simulink model "Power_Quality_Test2"  (R2015a)
settings: Solver=ode23t  StartTime=0.0  StopTime=0.5  RelTol=1e-5  AbsTol=1e-4
PreLoadFcn:
  | Ts=2e-6;
  | decimation = 1;
undefined symbols (not defined in the file or in its folder): HEV_Param
libraries: HEV_Electrical_Lib x5, fl_lib x2, simulink x1, HEV_Battery_Det_Lib x1, nesl_utility x1, powerlib x1
Description:
  | Copyright 2014 The MathWorks, Inc.
settings Model: CovSFcnEnable=off  Creator=smiller  LastModifiedBy=psanghvi
settings DataIOCC: SignalLoggingSaveFormat=ModelDataLogs
settings OptimizationCC: ExpressionDepthLimit=2147483647
settings DebuggingCC: UnderspecifiedInitializationDetection=Classic  MergeDetectMultiDrivingBlocksExec=none  SolverPrmCheckMsg=warning  FcnCallInpInsideContextMsg=UseLocalSettings  StateNameClashWarn=warning
settings SFSimCC: SimParseCustomCode=off
settings GRTTargetCC: CombineOutputUpdateFcns=off  GRTInterface=on

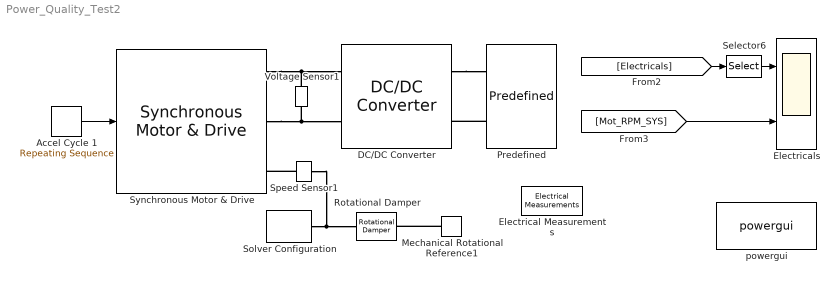
== system Power_Quality_Test2 ==
  Accel Cycle 1 : simulink/Sources/Repeating Sequence  rep_seq_t=[0 0.05 0.3 0.31 30]  rep_seq_y=[0 0.4 0.4 0.1 0.1]*100
  DC/DC Converter : HEV_Electrical_Lib/Detailed/DC//DC Converter  SystemSampleTime=-1
  Electrical Measurements : HEV_Electrical_Lib/Detailed/Electrical Measurements
  Electricals : Scope  NumInputPorts=2
      settings: YMin=499~200  YMax=501~500  SaveName=Electricals  Decimation=decimation
  Mechanical Rotational Reference1 : fl_lib/Mechanical/Rotational Elements/Mechanical Rotational Reference
  Predefined : HEV_Battery_Det_Lib/Predefined  SystemSampleTime=-1
  Rotational Damper : fl_lib/Mechanical/Rotational Elements/Rotational Damper  D=HEV_Param.ICE.Friction N*m/(rad/s)  w_specify=off  w_priority=High  w=0 rad/s  t_specify=off  t_priority=High  t=0 N*m
  Selector6 : Selector  InputPortWidth=8  Indices=[3 4]
  Solver Configuration : nesl_utility/Solver Configuration  PhysicalDomain=network_engine_domain  SubClassName=solver  LeftPortType=input  RightPortType=generic  Accelerate=off  Tones=[]  Harmonics=[]  SimulateNoise=off  Profile=off  UseLocalSampling=off  EnableSwitchedLinearOptims=on  FrequencyDomain=off  UseCCode=off  RelTol=0.001  AbsTol=1e-06  MinStep=1e-09  ToWorkspace=off  RevertToSquareIcSolve=off  NumHomotopyIterations=100  DoDC=off  ResidualTolerance=1e-9  UseLocalSolver=off  LocalSolverChoice=NE_BACKWARD_EULER_ADVANCER  LocalSolverSampleTime=.001  DoFixedCost=off  MaxNonlinIter=3  MaxModeIter=2  LinearAlgebra=Sparse  DelaysMemoryBudget=1024  AutomaticFiltering=on  FilteringTimeConstant=0.001
  Speed Sensor1 : HEV_Electrical_Lib/Detailed/Speed Sensor1  SystemSampleTime=-1
  Synchronous Motor & Drive : HEV_Electrical_Lib/Detailed/Synchronous Motor & Drive  SystemSampleTime=-1
  Voltage Sensor1 : HEV_Electrical_Lib/Detailed/Voltage Sensor1
  powergui : powerlib/powergui  SimulationMode=Discrete  SolverType=Tustin  SampleTime=Ts  frequency=60  SPID=on  DisableSnubberDevices=off  DisableRonSwitches=off  DisableVfSwitches=off  SwTol=0  DisplayEquations=off  Interpol=off  methode=off  Ts=0  FunctionMessages=off  echomessages=off  HookPort=off  EnableUseOfTLC=off  x0status=blocks  frequencyindice=0  Pbase=100e6  ErrMax=1e-4  Iterations=50  UnitsV=kV  UnitsW=MW  buscounter=0  RestoreLinks=warning  ResistiveCurrentMeasurement=off  Frange=[0:2:500]  Ylog=off  Xlog=on  ShowGrid=off  save=off  variable=ZData  structure=0  ZoomFFT=on  StartTime=0.0  cycles=1  DisplayStyle=1  fundamental=60  FreqAxis=off  MaxFrequency=1000  frequencyindicesteady=1  RmsSteady=1  display=off
  wires:
  [Electricals] -> Selector6/1
  Selector6/1 -> Electricals/1
  [Mot_RPM_SYS] -> Electricals/2
  Accel Cycle 1/1 -> Synchronous Motor & Drive/1
  connections:
  DC/DC Converter/LConn1 -- Predefined/LConn1
  Predefined/LConn2 -- DC/DC Converter/LConn2
  Synchronous Motor & Drive/RConn1 -- DC/DC Converter/RConn1 -- Voltage Sensor1/RConn1
  Synchronous Motor & Drive/RConn2 -- DC/DC Converter/RConn2 -- Voltage Sensor1/LConn1
  Solver Configuration/RConn1 -- Rotational Damper/LConn1 -- Speed Sensor1/RConn1
  Speed Sensor1/LConn1 -- Synchronous Motor & Drive/RConn3
  Mechanical Rotational Reference1/LConn1 -- Rotational Damper/RConn1
